simulink model "KF_tutorial"  (R2021a)
settings: Solver=VariableStepAuto  StartTime=0.0  StopTime=100  RelTol=1e-3
undefined symbols (not defined in the file): Continuous, Time
libraries: ctrlSharedLib x1
settings Model: Creator=giulio  LastModifiedBy=giulio
settings DebuggingCC: UnderSpecifiedDimensionMsg=warning

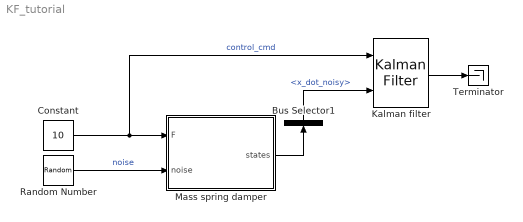
== system KF_tutorial ==
  Bus Selector1 : BusSelector  OutputSignals=x_dot_noisy
  Constant : Constant  Value=10
  "Kalman filter " : ctrlSharedLib/Kalman Filter  TimeDomain=Continuous-Time  UseCurrentEstimator=on  ModelSource=Individual A, B, C, D matrices  ModelSourceVariable=ss(0.95,1,1,0,1)  A=[0 1; -1/5 -0.6/5]  B=[0 1/5]'  C=[ 0 1]  D=0  NumberOfStates=2  NumberOfInputs=1  NumberOfOutputs=1  InitialEstimateSource=Dialog  X0=0  P0=10  UseK=off  UseGH=off  NumberOfProcessNoiseInputs=1  G=1  TimeInvariantG=on  H=0  TimeInvariantH=on  Q=0.05  TimeInvariantQ=on  R=0.6  TimeInvariantR=on  N=0  TimeInvariantN=on  AddInputPort=on  AddEnablePort=off  OutputEstimatedY=off  OutputP=off  Ts=-1
  Mass spring damper : Subsystem
  Random Number : RandomNumber  SampleTime=0.1
  Terminator : Terminator
  wires:
  Constant/1 -> Mass spring damper/1(F), "Kalman filter "/1  "control_cmd"
  Random Number/1 -> Mass spring damper/2(noise)  "noise"
  Mass spring damper/1(states) -> Bus Selector1/1
  Bus Selector1/1 -> "Kalman filter "/2  "<x_dot_noisy>"
  "Kalman filter "/1 -> Terminator/1

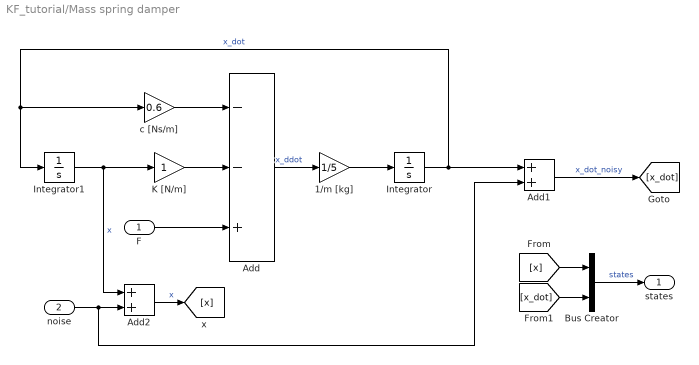
== system KF_tutorial/Mass spring damper ==
  F : Inport
  noise : Inport  Port=2
  1/m [kg] : Gain  Gain=1/5
  Add : Sum  Inputs=--+
  Add1 : Sum
  Add2 : Sum
  Bus Creator : BusCreator  Inputs=2
  Integrator : Integrator
  Integrator1 : Integrator
  K [N/m] : Gain
  c [Ns/m] : Gain  Gain=0.6
  states : Outport
  wires:
  F/1 -> Add/3
  1/m [kg]/1 -> Integrator/1
  Integrator1/1 -> Add2/1, K [N/m]/1  "x"
  c [Ns/m]/1 -> Add/1
  K [N/m]/1 -> Add/2
  Integrator/1 -> c [Ns/m]/1, Integrator1/1, Add1/1  "x_dot"
  Add/1 -> 1/m [kg]/1  "x_ddot"
  noise/1 -> Add1/2, Add2/2
  Bus Creator/1 -> states/1  "states"
  Add1/1 -> [x_dot]  "x_dot_noisy"
  Add2/1 -> [x]  "x"
  [x] -> Bus Creator/1
  [x_dot] -> Bus Creator/2
